simulink model "MotorControlLibNEWFixedP_FULL19b"  (R2020b)
settings: Solver=FixedStepDiscrete  StartTime=0.0  StopTime=100  FixedStep=Ts  RelTol=1e-3
values from neighbouring files (symbols this model uses):
  Ki_Iab_EMFobs = 1600.0    [MotorControl.sldd]
  Kp_Iab_EMFobs = 0.255    [MotorControl.sldd]
  p = 8/2    (= 4)    [MotorControlLibData.m]    (also in local_pmsm_torque_control_data.m = 8)
  Ts = 250.0e-06    (= 0.00025)    [MotorControlLibData.m]    (also in local_pmsm_torque_control_data.m = 5e-06)
undefined symbols (not defined in the file or in its folder): BrkPoints, CuttOffFreq_c, d_q_Voltage_Limiter_max, d_q_Voltage_Limiter_sat_neg, d_q_Voltage_Limiter_sat_pos, DiscIntNeverNeededParam, Down, dSoll, EMFobsLdGain, EMFobsRS, Ki_dAxis, Ki_qAxis, Kp_dAxis, Kp_qAxis, MaxBckEMFVol_sat_neg, MaxBckEMFVol_sat_pos, NumBits1, NumBits2, pwmTableData, qSoll, Slope1, Slope2, TqToIqConst, TsIntern, Up
libraries: simulink x13, pid_lib x6, eePwmGenerator x3, simulink_extras x2
(part 1 of 3)
settings Model: DataDictionary=MotorControl.sldd  NumberOfSteps=10  Creator=unix  LastModifiedBy=unix
settings SolverCC: AutoInsertRateTranBlk=on
settings OptimizationCC: DefaultParameterBehavior=Inlined  EnhancedBackFolding=on  PassReuseOutputArgsAs=Individual arguments  ZeroExternalMemoryAtStartup=off  ZeroInternalMemoryAtStartup=off  OptimizeBlockOrder=speed  DifferentSizesBufferReuse=on  OptimizationCustomize=off  EfficientTunableParamExpr=on
settings DebuggingCC: ArrayBoundsChecking=warning  SignalInfNanChecking=warning  SignalRangeChecking=warning  CheckMatrixSingularityMsg=warning  IntegerOverflowMsg=error  ParameterOverflowMsg=warning  ParameterUnderflowMsg=warning  ParameterPrecisionLossMsg=none  ParameterTunabilityLossMsg=error  UnderSpecifiedDataTypeMsg=warning  IntegerSaturationMsg=error
settings SFSimCC: MATLABDynamicMemAlloc=off
settings RTWCC: Description=Embedded Coder  SystemTargetFile=ert.tlc  GenCodeOnly=on  TemplateMakefile=ert_default_tmf  GenerateReport=on  IncludeHyperlinkInReport=on  LaunchReport=on  GenerateTraceInfo=on  GenerateTraceReport=on  GenerateTraceReportSl=on  GenerateTraceReportSf=on  GenerateTraceReportEml=on
settings CodeAppCC: ForceParamTrailComments=on  IgnoreCustomStorageClasses=off  OperatorAnnotations=on  SimulinkDataObjDesc=on  SFDataObjDesc=on  InsertBlockDesc=on
settings ERTTargetCC: TargetLangStandard=C99 (ISO)  GenerateSampleERTMain=on  GenerateASAP2=on  InlinedParameterPlacement=NonHierarchical  ERTCustomFileTemplate=example_file_process.tlc

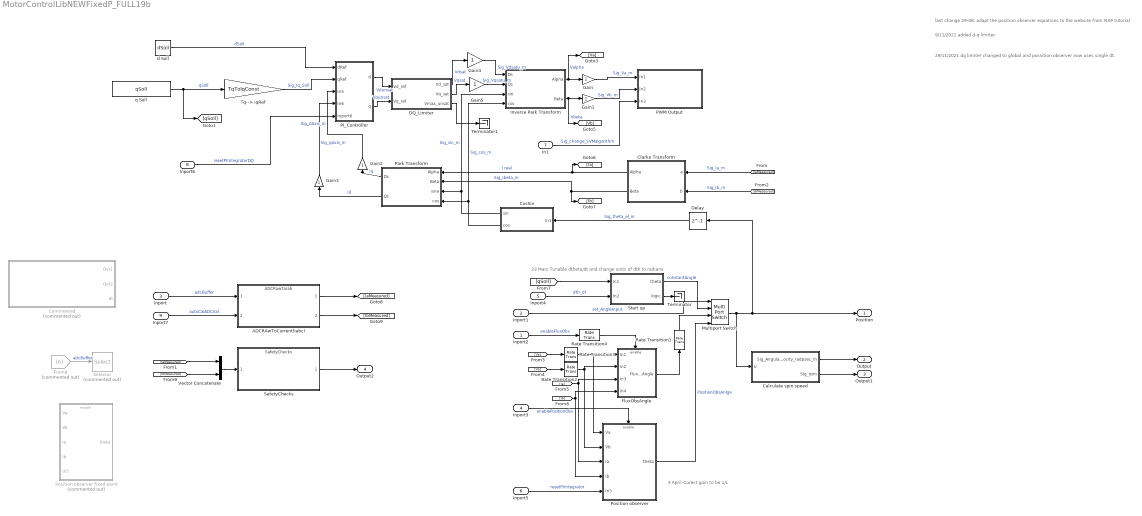
== system MotorControlLibNEWFixedP_FULL19b ==
  note: 29/11/2021 dq limiter changed to global and possition observer now uses single dt.
  note: 9/11/2021 added d-q limiter.
  note: last change 29-08: adapt the position observer equations to the website from NXP tutorial
  note: 3 April-Corect gain to be 1/L
  note: 23 Marz Tunable dtheta/dt and change units of dth to radians
  Inport2 : Inport  OutDataTypeStr=boolean  SampleTime=4*Ts
      settings: AttributesFormatString=%<SampleTime>
  Inport1 : Inport  Port=2  OutDataTypeStr=uint8  SampleTime=4*Ts
      settings: AttributesFormatString=%<SampleTime>
  Inport : Inport  Port=3
  Inport3 : Inport  Port=4  OutDataTypeStr=boolean  SampleTime=4*Ts
      settings: AttributesFormatString=%<SampleTime>
  Inport4 : Inport  Port=5
  Inport5 : Inport  Port=6  OutDataTypeStr=boolean  SampleTime=4*Ts
      settings: AttributesFormatString=%<SampleTime>
  In1 : Inport  Port=7
  Inport6 : Inport  Port=8  OutDataTypeStr=boolean
  Inport7 : Inport  Port=9
  ADCRAwToCurrent(Iabc) : ModelReference  ModelNameDialog=ADCRawToIab  ModelReferenceVersion=3.5
  Calculate spin speed : Subsystem  TreatAsAtomicUnit=on  SystemSampleTime=4*Ts
  Clarke Transform : Subsystem  VariantControl=Variant2  mask(Clarke Transform){}
      mask help:
      | <p>Compute Clarke transformation on balanced 3-phase inputs into balanced 2-phase orthogonal outputs.
      | <br>
      | <br>
      | The block accepts two signals out of three phases, and outputs corresponding &alpha;-&beta; axis components, where phase-a axis is aligned with alpha axis.</p>
      mask Help: eval('mcb.internal.helpview(''clarketransform'')')
      mask Display: mcb.internal.drawIcons('Clarke',1);
  Commented : Subsystem  Commented=on
  CosSin : Subsystem
  DQ_Limiter : Subsystem  TreatAsAtomicUnit=on  SystemSampleTime=4*Ts  mask(DQ Limiter){Vmax=d_q_Voltage_Limiter_max}
      mask prompts: Vmax "D-Q saturation limit:"
      mask help:
      | Implement saturation on reference dq voltages, with respect to phase voltage peak limit.
      |
      | The block accepts reference values of d and q axis voltages, and outputs corresponding saturated values along with unsaturated peak value to initiate field weakening control.
      |
      | Enter the phase voltage peak limit in the dialog box to initiate saturation.
      settings: RTWFcnNameOpts=Use subsystem name
      mask Help: eval('mcb.internal.helpview(''dqlimiter'')')
  Delay : Delay  DelayLength=1  SampleTime=4*Ts
      settings: AttributesFormatString=%<SampleTime>
  FluxObsAngle : Subsystem
      settings: RTWFcnNameOpts=Use subsystem name
  From8 : From  Commented=on
  Gain{,1..3} (4 alike) : Gain  OutDataTypeStr=Inherit: Same as input  ParamDataTypeStr=Inherit: Same as input
  Gain4 : Gain  OutDataTypeStr=Inherit: Inherit via back propagation
  Gain5 : Gain  OutDataTypeStr=Inherit: Inherit via back propagation
  Inverse Park Transform : Subsystem  SystemSampleTime=250*Ts  mask(Inverse Park Transform){AxisAlignment=D-axis}
      mask prompts: AxisAlignment "Alpha (phase-a) axis alignment:"
      mask help:
      | <p>Compute Inverse Park transformation on rotating reference frame inputs into stationary reference frame outputs.
      | <br><br>
      | The block accepts the following:
      | <ul>
      | <li>d-q axis components in rotating reference frame</li>
      | <li>Sine and cosine values of corresponding angle of transformation</li>
      | </ul>
      | The block outputs &alpha;-&beta; axis components in stationary reference frame.
      | <br><br>
      | D-axis alignment with alpha (phase-a) is popular in motor control theory while Q-axis alignment with alpha (phase-a) is more suitable for power conversion applications.</p>
      mask Help: eval('mcb.internal.helpview(''inverseparktransform'')')
      mask TypeOptions AxisAlignment: D-axis | Q-axis
  Multiport Switch : MultiPortSwitch  DataPortOrder=Zero-based contiguous  zeroidx=on
  PI_Controller : Subsystem  TreatAsAtomicUnit=on  SystemSampleTime=4*Ts
      settings: RTWFcnNameOpts=Use subsystem name
  PWM Output : Subsystem
  Park Transform : Subsystem  SystemSampleTime=250*Ts  mask(Park Transform){AxisAlignment=D-axis}
      mask prompts: AxisAlignment "Alpha (phase-a) axis alignment:"
      mask help:
      | <p>Compute Park transformation on stationary reference frame inputs into rotating reference frame outputs.
      | <br><br>
      | The block accepts the following:
      | <ul>
      |   <li>&alpha;-&beta; axis components in stationary reference frame</li>
      |   <li>Sine and cosine values of corresponding angle of transformation</li>
      | </ul>
      | The block outputs direct and quadrature axis components in rotating reference frame.
      | <br><br>
      | D-axis alignment with alpha (phase-a) is popular in motor control theory while Q-axis alignment with alpha (phase-a) is more suitable for power conversion applications.</p>
      mask Help: eval('mcb.internal.helpview(''parktransform'')')
      mask TypeOptions AxisAlignment: D-axis | Q-axis
      mask Display: mcb.internal.drawIcons('Park',1);
  Position observer : Subsystem
  Position observer fixed point : Subsystem  Commented=on
  Rate Transition{1..4} (4 alike) : RateTransition
  SafetyChecks : ModelReference  ModelNameDialog=SafetyChecks.slx  ModelReferenceVersion=1.11
  Selector : Selector  Commented=on  InputPortWidth=3  IndexOptions=Index vector (dialog)  Indices=[1 2]  OutputSizes=1
  Start up : Subsystem  TreatAsAtomicUnit=on  SystemSampleTime=4*Ts
  Terminator : Terminator
  Terminator1 : Terminator
  Tq--> iqRef : Gain  Gain=TqToIqConst  ParamDataTypeStr=Inherit: Inherit from 'Gain'  OutDataTypeStr=fixdt(1,16,2^-8,0)
  Vector Concatenate : Concatenate
  d Soll : Constant  Value=dSoll
  q Soll : Constant  Value=qSoll
  Position : Outport
  Output : Outport  Port=2
  Output1 : Outport  Port=3  Unit=rpm
  Output2 : Outport  Port=4
  wires:
  [IbMeasured] -> Clarke Transform/2(b)  "Sig_Ib_m"
  [IaMeasured] -> Clarke Transform/1(a)  "Sig_Ia_m"
  Clarke Transform/1(Alpha) -> [Ia], Park Transform/1(Alpha)  "I real"
  Clarke Transform/2(Beta) -> [Ib], Park Transform/2(Beta)  "Sig_Ibeta_m"
  Inverse Park Transform/1(Alpha) -> [Va], Gain/1  "Valpha"
  Gain4/1 -> Inverse Park Transform/1(Ds)  "Sig_Vdsatu_m"
  Gain5/1 -> Inverse Park Transform/2(Qs)  "Sig_Vqsatu_m"
  Inverse Park Transform/2(Beta) -> Gain1/1, [Vb]  "Vbeta"
  d Soll/1 -> PI_Controller/1(dRef)  "dSoll"
  Tq--> iqRef/1 -> PI_Controller/2(qRef)  "Sig_Iq_Soll"
  PI_Controller/1(d) -> DQ_Limiter/1(Vd_ref)  "Vdunsat"
  PI_Controller/2(q) -> DQ_Limiter/2(Vq_ref)  "Vqunsat"
  Park Transform/2(Qs) -> Gain3/1  "Id"
  Park Transform/1(Ds) -> Gain2/1  "Iq"
  q Soll/1 -> [qSoll], Tq--> iqRef/1  "qSoll"
  ADCRAwToCurrent(Iabc)/2 -> [IbMeasured]
  Inport/1 -> ADCRAwToCurrent(Iabc)/1  "adcBuffer"
  ADCRAwToCurrent(Iabc)/1 -> [IaMeasured]
  CosSin/1(sin) -> Inverse Park Transform/3(sin), Park Transform/3(sine)  "Sig_sin_m"
  CosSin/2(cos) -> Park Transform/4(cos), Inverse Park Transform/4(cos)  "Sig_cos_m"
  Delay/1 -> CosSin/1(In1)  "Sig_theta_el_m"
  Gain/1 -> PWM Output/1(In1)  "Sig_Va_m"
  Gain1/1 -> PWM Output/2(In2)  "Sig_Vb_m"
  Gain2/1 -> PI_Controller/3(In5)  "Sig_dAxis_m"
  Gain3/1 -> PI_Controller/4(In6)  "Sig_qAxis_m"
  [qSoll] -> Start up/1(In1)
  Start up/1(theta) -> Multiport Switch/2  "constantAngle"
  Start up/2(logic) -> Terminator/1
  Inport1/1 -> Multiport Switch/1  "set_AngleInput"
  FluxObsAngle/1(FluxObsAngle) -> Rate Transition1/1
  Inport2/1 -> Rate Transition4/1  "enableFluxObs"
  Inport3/1 -> Position observer/Enable  "enablePositionObs"
  Position observer/1(theta) -> Multiport Switch/4  "PositionObsAnlge"
  Rate Transition2/1 -> FluxObsAngle/2(In2), Position observer/2(Vb)
  Rate Transition3/1 -> Position observer/1(Va), FluxObsAngle/1(In1)
  [Ia] -> FluxObsAngle/3(In3), Position observer/3(Ia)
  [Ib] -> FluxObsAngle/4(In4), Position observer/4(Ib)
  From8/1 -> Selector/1  "adcBuffer"
  Inport4/1 -> Start up/2(In2)  "dth_dt"
  Inport5/1 -> Position observer/5(In5)  "resetPIIntegrator"
  DQ_Limiter/2(Vq_sat) -> Gain5/1  "Vqsat"
  DQ_Limiter/1(Vd_sat) -> Gain4/1  "Vdsat"
  DQ_Limiter/3(Vmax_unsat) -> Terminator1/1
  Rate Transition4/1 -> FluxObsAngle/Enable
  In1/1 -> PWM Output/3(In3)  "Sig_change_SVMalgorithm"
  Multiport Switch/1 -> Calculate spin speed/1(U), Delay/1, Position/1
  Inport6/1 -> PI_Controller/5(Inport6)  "resetPIIntegratorDQ"
  Rate Transition1/1 -> Multiport Switch/3
  [Vb] -> Rate Transition2/1
  [Va] -> Rate Transition3/1
  Calculate spin speed/1(Sig_Angular_Velocity_radpsec_m) -> Output/1
  Calculate spin speed/2(Sig_rpm) -> Output1/1
  Vector Concatenate/1 -> SafetyChecks/1
  [IaMeasured] -> Vector Concatenate/1
  [IbMeasured] -> Vector Concatenate/2
  SafetyChecks/1 -> Output2/1
  Inport7/1 -> ADCRAwToCurrent(Iabc)/2  "autoCalADCVal"

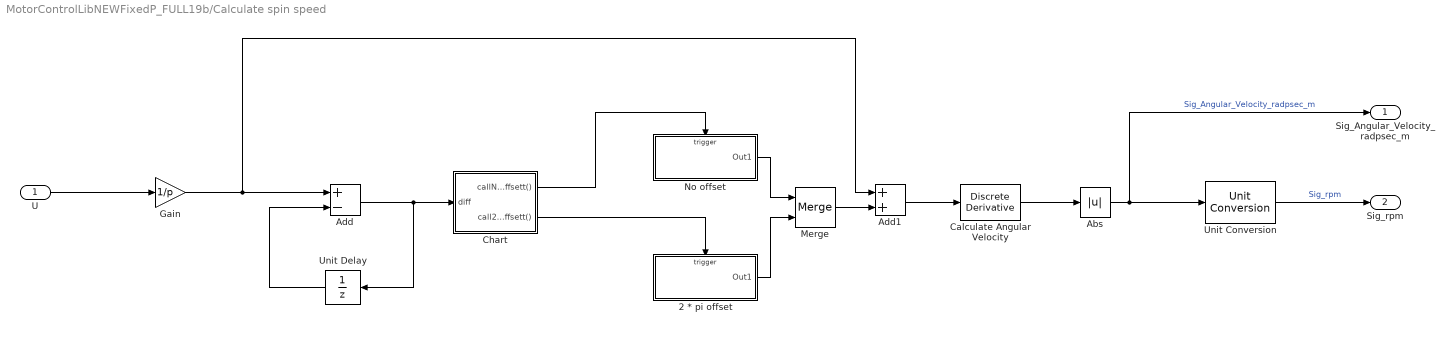
== system MotorControlLibNEWFixedP_FULL19b/Calculate spin speed ==
  U : Inport
  2 * pi offset : Subsystem  TreatAsAtomicUnit=on
  Abs : Abs
  Add : Sum  Inputs=+-
  Add1 : Sum
  Calculate Angular Velocity : simulink/Discrete/Discrete Derivative  gainval=1.0  ICPrevScaledInput=0.0  OutMin=[]  OutMax=[]  OutDataTypeStr=single  OutputDataTypeScalingMode=single  OutDataType=fixdt(1, 16)  OutScaling=2^-10  DoSatur=off
  Chart : Stateflow chart  TreatAsAtomicUnit=on
  Gain : Gain  Gain=1/p  OutDataTypeStr=single
  Merge : Merge
  No offset : Subsystem  TreatAsAtomicUnit=on
  Unit Conversion : UnitConversion
  Unit Delay : UnitDelay  SampleTime=-1  HasFrameUpgradeWarning=on
  Sig_Angular_Velocity_radpsec_m : Outport
  Sig_rpm : Outport  Port=2
  wires:
  U/1 -> Gain/1
  Unit Conversion/1 -> Sig_rpm/1  "Sig_rpm"
  Abs/1 -> Unit Conversion/1, Sig_Angular_Velocity_radpsec_m/1  "Sig_Angular_Velocity_radpsec_m"
  Calculate Angular Velocity/1 -> Abs/1
  Unit Delay/1 -> Add/2
  Add/1 -> Unit Delay/1, Chart/1(diff)
  Chart/2(call2PiOffsett()) -> 2 * pi offset/Trigger
  Chart/1(callNoOffsett()) -> No offset/Trigger
  2 * pi offset/1(Out1) -> Merge/2
  No offset/1(Out1) -> Merge/1
  Merge/1 -> Add1/2
  Add1/1 -> Calculate Angular Velocity/1
  Gain/1 -> Add1/1, Add/1

== system MotorControlLibNEWFixedP_FULL19b/Clarke Transform ==
  a : Inport
  b : Inport  Port=2
  Data Type Duplicate : DataTypeDuplicate
  a_plus_2b : Sum  Inputs=+++  RndMeth=Simplest  OutDataTypeStr=Inherit: Same as first input
  one_by_sqrt3 : Gain  Gain=1/sqrt(3)  RndMeth=Simplest  OutDataTypeStr=Inherit: Same as input
  Alpha : Outport  VectorParamsAs1DForOutWhenUnconnected=off
  Beta : Outport  Port=2  VectorParamsAs1DForOutWhenUnconnected=off
  wires:
  a/1 -> a_plus_2b/1, Alpha/1, Data Type Duplicate/1
  one_by_sqrt3/1 -> Beta/1
  a_plus_2b/1 -> one_by_sqrt3/1
  b/1 -> a_plus_2b/2, a_plus_2b/3, Data Type Duplicate/2

== system MotorControlLibNEWFixedP_FULL19b/Commented ==
  Digital Clock : DigitalClock  Commented=on  SampleTime=Ts
  Function-Call Clock_50us : simulink/Ports & Subsystems/Function-Call Generator  Commented=on  sample_time=5e-5  numberOfIterations=1  DisallowWideOutput=off
  Function-Call Clock_50us1 : simulink/Ports & Subsystems/Function-Call Generator  Commented=on  sample_time=Ts  numberOfIterations=1  DisallowWideOutput=off
  Function-Call Split : FunctionCallSplit  Commented=on  IconShape=distinctive  NumOutputPorts=3  OutputPortLayout=default
  Goto1 : Goto  Commented=on  GotoTag=Task100us_2
  Goto2 : Goto  Commented=on  GotoTag=Task100us_1
  Goto4 : Goto  Commented=on  GotoTag=Task1ms_1
  Rate Transition8 : RateTransition  Commented=on
  Subsystem : Subsystem  Commented=on
  Task Scheduler : Stateflow chart  Commented=on  TreatAsAtomicUnit=on
  Out1 : Outport
  Out2 : Outport  Port=2
  dt : Outport  Port=3
  wires:
  Task Scheduler/2(Task_100us_2()) -> Goto1/1
  Function-Call Clock_50us/1 -> Task Scheduler/Trigger
  Digital Clock/1 -> Rate Transition8/1
  Rate Transition8/1 -> Subsystem/1(Clock)
  Function-Call Clock_50us1/1 -> Function-Call Split/1
  Function-Call Split/3 -> Subsystem/Trigger
  Subsystem/1(dt) -> dt/1
  Function-Call Split/2 -> Out2/1
  Function-Call Split/1 -> Out1/1
  Task Scheduler/1(Task_100us_1()) -> Goto2/1
  Task Scheduler/3(Task_1ms_1()) -> Goto4/1

== system MotorControlLibNEWFixedP_FULL19b/CosSin ==
  In1 : Inport
  Data Type Conversion1 : DataTypeConversion
  Sine-Cosine Lookup : Subsystem  mask(Sine-Cosine Lookup){AngleInput=Radians, N_points=512}
      mask prompts: AngleInput "Theta units:"; N_points "Number of data points for lookup table:"
      mask help:
      | Implement sine and cosine functions using a lookup table approach for optimized performance on target hardware.
      |
      | The block accepts input angle in different units and outputs corresponding sine and cosine values.
      mask init:
      | % dlgSett = mct.internal.SinCosCb(gcbh);
      | this = get_param(gcbh,'Object');
      | 
      | points = eval(this.N_points);
      | 
      | dlgSett.points = 125*floor(points/125);
      | 
      | dlgSett.Offset = uint16(dlgSett.points/5);
      | 
      | dlgSett.N_points = 4*dlgSett.Offset;
      | N_points = dlgSett.N_points;
      | 
      | theta = linspace(0,2*pi,N_points+1);
      | dlgSett.size = 5*dlgSett.Offset+2;
      | dlgSett.sin_table = zeros(1,dlgSett.size);
      | dlgSett.sin_table(1:N_points+1) = sin(theta);
      | dlgSett.sin_table(N_points+2:dlgSett.size) = dlgSett.sin_table(2:0.25*N_points+2);
      | 
      | dlgSett.N_points = double(dlgSett.N_points);
      | dlgSett.index_gain = dlgSett.N_points;
      | dlgSett.UpperSatLimit = 1;
      | 
      | switch AngleInput
      |     case 1
      |         dlgSett.UpperSatLimit = 1;
      |     case 2
      |         dlgSett.UpperSatLimit = 2*pi;
      |     case 3
      |         dlgSett.UpperSatLimit = 360;
      |     otherwise
      | end
      mask Help: eval('mcb.internal.helpview(''sinecosinelookup'')')
      mask TypeOptions AngleInput: Per-unit | Radians | Degrees
      mask Display: mcb.internal.drawIcons('Sin-Cos',1);
  sin : Outport
  cos : Outport  Port=2
  wires:
  Sine-Cosine Lookup/2(cos) -> cos/1
  In1/1 -> Data Type Conversion1/1
  Sine-Cosine Lookup/1(sin) -> sin/1
  Data Type Conversion1/1 -> Sine-Cosine Lookup/1(Theta)

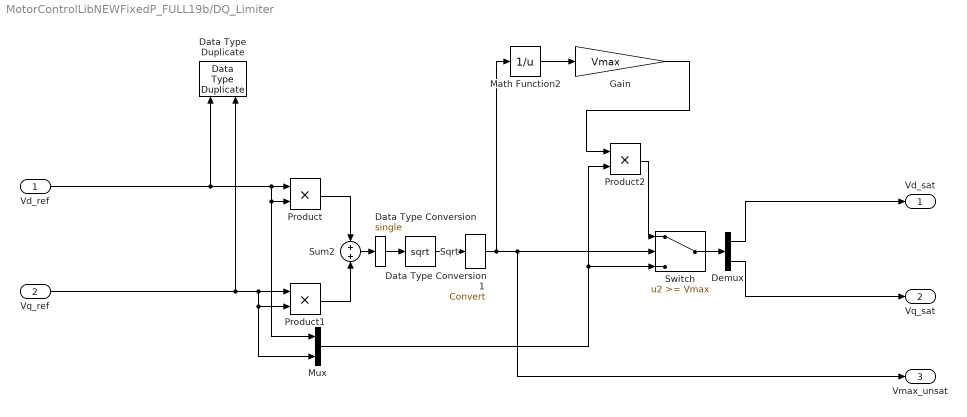
== system MotorControlLibNEWFixedP_FULL19b/DQ_Limiter ==
  Vd_ref : Inport
  Vq_ref : Inport  Port=2
  Data Type Duplicate : DataTypeDuplicate
  Data Type Conversion : DataTypeConversion  OutDataTypeStr=single
  Data Type Conversion1 : DataTypeConversion
  Demux : Demux  Outputs=2
  Gain : Gain  Gain=Vmax  OutDataTypeStr=Inherit: Same as input
  Math Function2 : Math  Operator=reciprocal  SignedPower=on  RndMeth=Simplest
  Mux : Mux  Inputs=2
  Product : Product  RndMeth=Simplest  OutDataTypeStr=Inherit: Same as first input
  Product1 : Product  RndMeth=Simplest  OutDataTypeStr=Inherit: Same as first input
  Product2 : Product  OutDataTypeStr=Inherit: Same as first input
  Sqrt : Sqrt  IntermediateResultsDataTypeStr=Inherit: Inherit from input  SaturateOnIntegerOverflow=on
  Sum2 : Sum  OutDataTypeStr=Inherit: Same as first input
  Switch : Switch  Threshold=Vmax  ZeroCross=off
  Vd_sat : Outport  VectorParamsAs1DForOutWhenUnconnected=off
  Vq_sat : Outport  Port=2  VectorParamsAs1DForOutWhenUnconnected=off
  Vmax_unsat : Outport  Port=3  VectorParamsAs1DForOutWhenUnconnected=off
  wires:
  Vd_ref/1 -> Data Type Duplicate/1, Product/1, Product/2, Mux/1
  Demux/1 -> Vd_sat/1
  Product1/1 -> Sum2/2
  Product/1 -> Sum2/1
  Sum2/1 -> Data Type Conversion/1
  Math Function2/1 -> Gain/1
  Mux/1 -> Product2/2, Switch/3
  Product2/1 -> Switch/1
  Switch/1 -> Demux/1
  Demux/2 -> Vq_sat/1
  Sqrt/1 -> Data Type Conversion1/1
  Gain/1 -> Product2/1
  Vq_ref/1 -> Data Type Duplicate/2, Product1/1, Product1/2, Mux/2
  Data Type Conversion1/1 -> Vmax_unsat/1, Switch/2, Math Function2/1
  Data Type Conversion/1 -> Sqrt/1

== system MotorControlLibNEWFixedP_FULL19b/FluxObsAngle ==
  In1 : Inport
  In2 : Inport  Port=2
  In3 : Inport  Port=3
  In4 : Inport  Port=4
  Enable : EnablePort
  Flux Observer : Subsystem  TreatAsAtomicUnit=on  SystemSampleTime=2*Ts  mask(Flux Observer){BlockInputUnit=SI unit, PerUnitVoltage=13.86, PerUnitCurrent=19.3, PositionSelect=on, FluxSelect=off, TorqueSelect=off, PolePairs=4, StatorResistance=EMFobsRS, StatorDAxisInductance=EMFobsLdGain, BlockSampleTime=2*Ts, PositionUnit=Radians, PositionDatatype=fixdt(1,16,2^-8,0), FluxUnit=Weber, PerUnitFlux=0.1, FluxDatatype=single, TorqueUnit=Nm, PerUnitTorque=100, TorqueDatatype=single}
      mask prompts: BlockInputUnit "Input units:"; PerUnitVoltage "Per unit reference voltage (V):"; PerUnitCurrent "Per unit reference current (A):"; PositionSelect "Position"; FluxSelect "Flux"; TorqueSelect "Torque"; PolePairs "Pole pairs:"; StatorResistance "Stator resistance (ohm):"; StatorDAxisInductance "Stator d-axis inductance (H):"; BlockSampleTime "Block sample time (S):"; PositionUnit "Position unit:"; PositionDatatype "Position datatype:"; FluxUnit "Flux unit:"; PerUnitFlux "Per unit flux (Wb):"; FluxDatatype "Flux datatype:"; TorqueUnit "Torque unit:"; PerUnitTorque "Per unit torque (Nm):"; TorqueDatatype "Torque datatype:"
      mask help:
      | <p>Compute &#952;<sub>e</sub> (electrical position), &#936; (magnetic flux), and T<sub>e</sub> (electrical torque) of a PMSM from the measured voltage and current in the stationary reference frame.
      | <br><br>
      | Use the Input units parameter to select the input unit of the block.
      | <br><br>
      | Use the Per unit reference voltage parameter to enter the amplitude of line-to-neutral voltage used as a reference. Use the Per unit reference current parameter to enter the amplitude of line current used as a reference.</P>
      mask init:
      | %mcb.internal.FOCb('MaskInitFcn', gcbh);
      mask Help: eval('mcb.internal.helpview(''fluxobserver'')')
      mask TypeOptions BlockInputUnit: SI unit | Per-unit
      mask Callback BlockInputUnit: mcb.internal.FOCb('MaskDisplay', gcbh);
      mask Callback PositionSelect: mcb.internal.FOCb('MaskDisplay', gcbh);
      mask Callback FluxSelect: mcb.internal.FOCb('MaskDisplay', gcbh);
      mask Callback TorqueSelect: mcb.internal.FOCb('MaskDisplay', gcbh);
      mask TypeOptions PositionUnit: Radians | Degrees | Per-unit
      mask TypeOptions FluxUnit: Weber | Per-unit
      mask Callback FluxUnit: mcb.internal.FOCb('MaskDisplay', gcbh);
      mask TypeOptions TorqueUnit: Nm | Per-unit
      mask Callback TorqueUnit: mcb.internal.FOCb('MaskDisplay', gcbh);
      mask DialogControl Container4 Prompt: Motor Parameters
      mask DialogControl Container7 Prompt: Block Output
      mask DialogControl Container8 Prompt: Datatypes
      mask Display:
      | color('black');
      | port_label('input',1, 'V_{\alpha}', 'interpreter', 'tex');
      | port_label('input',2, 'V_{\beta}', 'interpreter', 'tex');
      | port_label('input',3, 'I_{\alpha}', 'interpreter', 'tex');
      | port_label('input',4, 'I_{\beta}', 'interpreter', 'tex');
      | port_label('input',5, 'Rst', 'interpreter', 'tex');
      | port_label('output',1, '\theta_{e}', 'interpreter', 'tex');
      | %No Flux;
      | %No Torque;
      | fprintf('Flux\nObserver');
  Ground : Ground
  FluxObsAngle : Outport
  wires:
  In1/1 -> Flux Observer/1(Valpha)
  Ground/1 -> Flux Observer/5(Reset)
  In4/1 -> Flux Observer/4(Ibeta)
  In2/1 -> Flux Observer/2(Vbeta)
  In3/1 -> Flux Observer/3(Ialpha)
  Flux Observer/1(Position) -> FluxObsAngle/1  "FluxObsAngle"

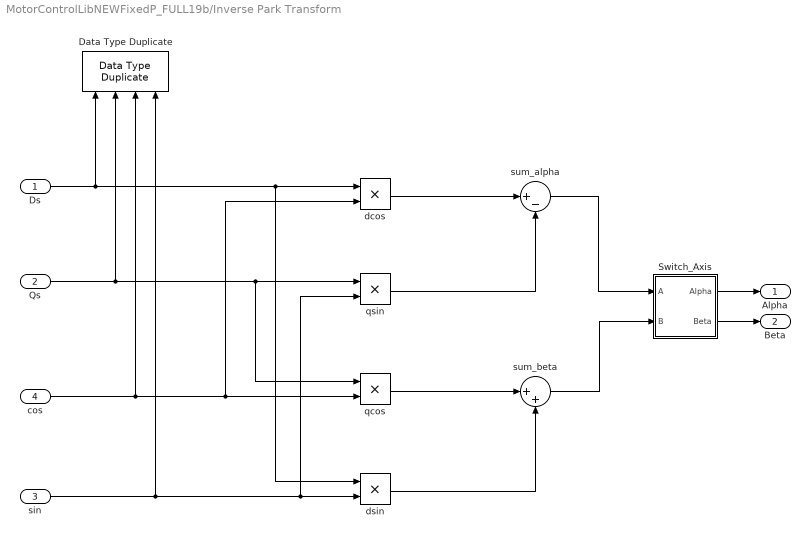
== system MotorControlLibNEWFixedP_FULL19b/Inverse Park Transform ==
  Ds : Inport
  Qs : Inport  Port=2
  sin : Inport  Port=3
  cos : Inport  Port=4
  Data Type Duplicate : DataTypeDuplicate  NumInputPorts=4
  Switch_Axis : Subsystem
  dcos : Product  RndMeth=Simplest  OutDataTypeStr=Inherit: Same as first input
  dsin : Product  RndMeth=Simplest  OutDataTypeStr=Inherit: Same as first input
  qcos : Product  RndMeth=Simplest  OutDataTypeStr=Inherit: Same as first input
  qsin : Product  RndMeth=Simplest  OutDataTypeStr=Inherit: Same as first input
  sum_alpha : Sum  Inputs=|+-  RndMeth=Simplest  OutDataTypeStr=Inherit: Same as first input
  sum_beta : Sum  Inputs=|++  RndMeth=Simplest  OutDataTypeStr=Inherit: Same as first input
  Alpha : Outport  VectorParamsAs1DForOutWhenUnconnected=off
  Beta : Outport  Port=2  VectorParamsAs1DForOutWhenUnconnected=off
  wires:
  Switch_Axis/2(Beta) -> Beta/1
  Switch_Axis/1(Alpha) -> Alpha/1
  sum_beta/1 -> Switch_Axis/2(B)
  sum_alpha/1 -> Switch_Axis/1(A)
  sin/1 -> dsin/2, qsin/2, Data Type Duplicate/4
  cos/1 -> qcos/2, dcos/2, Data Type Duplicate/3
  dsin/1 -> sum_beta/2
  Qs/1 -> qsin/1, qcos/1, Data Type Duplicate/2
  dcos/1 -> sum_alpha/1
  qcos/1 -> sum_beta/1
  qsin/1 -> sum_alpha/2
  Ds/1 -> dcos/1, dsin/1, Data Type Duplicate/1

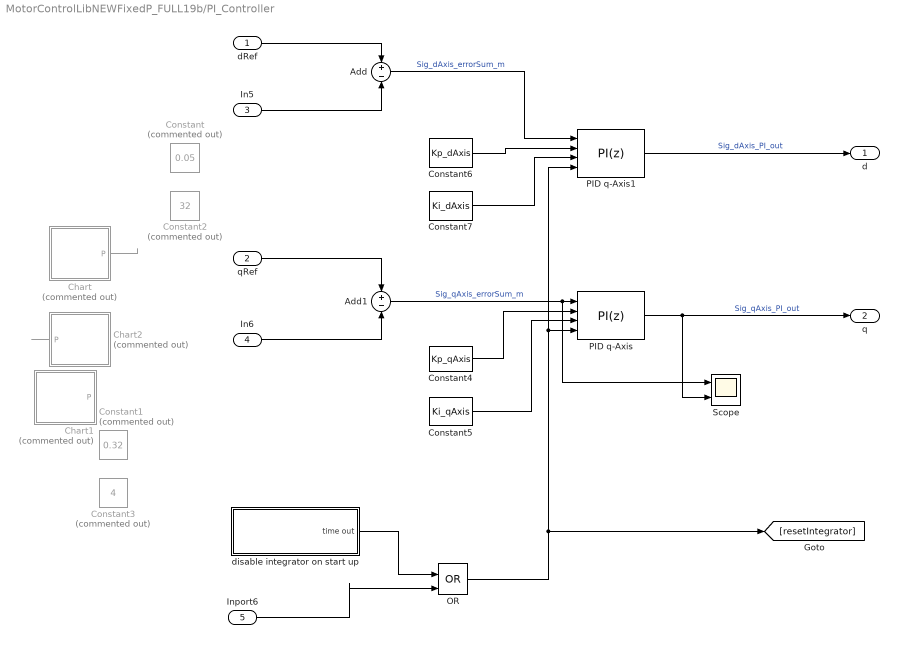
== system MotorControlLibNEWFixedP_FULL19b/PI_Controller ==
  dRef : Inport
  qRef : Inport  Port=2
  In5 : Inport  Port=3
  In6 : Inport  Port=4
  Inport6 : Inport  Port=5
  Add : Sum  Inputs=+|-
  Add1 : Sum  Inputs=+|-
  Chart : Stateflow chart  Commented=on  TreatAsAtomicUnit=on  SystemSampleTime=1000*Ts
  Chart1 : Stateflow chart  Commented=on  TreatAsAtomicUnit=on  SystemSampleTime=2000*Ts
  Chart2 : Stateflow chart  Commented=on  TreatAsAtomicUnit=on  SystemSampleTime=100000*Ts
  Constant : Constant  Commented=on  Value=0.05  OutDataTypeStr=fixdt(1,16,2^-7,0)
  Constant1 : Constant  Commented=on  Value=0.32  OutDataTypeStr=fixdt(1,8,2^-7,0)
  Constant2 : Constant  Commented=on  Value=32  OutDataTypeStr=fixdt(1,8,2^-1,0)
  Constant3 : Constant  Commented=on  Value=4  OutDataTypeStr=fixdt(1,8,2^-1,0)
  Constant4 : Constant  Value=Kp_qAxis
  Constant5 : Constant  Value=Ki_qAxis
  Constant6 : Constant  Value=Kp_dAxis
  Constant7 : Constant  Value=Ki_dAxis
  OR : Logic  Operator=OR  IconShape=distinctive  AllPortsSameDT=off  OutDataTypeStr=boolean
  PID q-Axis : pid_lib/PID Controller  Controller=PI  Form=Parallel  TimeDomain=Discrete-time  UseExternalTs=off  SampleTime=-1  IntegratorMethod=Forward Euler  FilterMethod=Forward Euler  ControllerParametersSource=external  P=0  I=0  D=0  UseFilter=on  N=100  TunerSelectOption=Transfer Function Based (PID Tuner App)  InitialConditionSource=internal  InitialConditionForIntegrator=0  InitialConditionForFilter=0  DifferentiatorICPrevScaledInput=0  ExternalReset=level  TrackingMode=off  Kt=1  LimitOutput=on  SatLimitsSource=internal  UpperSaturationLimit=d_q_Voltage_Limiter_sat_pos  LowerSaturationLimit=d_q_Voltage_Limiter_sat_neg  LinearizeAsGain=off  AntiWindupMode=clamping  Kb=10  PGainOutDataTypeStr=fixdt(1,16,2^-8,0)  PProdOutDataTypeStr=fixdt(1,16,2^-8,0)  POutMin=[]  POutMax=[]  IGainOutDataTypeStr=fixdt(1,16,2^-8,0)  IProdOutDataTypeStr=fixdt(1,16,2^-8,0)  IOutMin=[]  IOutMax=[]  DOutMin=[]  DOutMax=[]  NOutMin=[]  NOutMax=[]  SumOutDataTypeStr=fixdt(1,16,2^-8,0)  SumOutMin=[]  SumOutMax=[]  SaturationOutMin=[]  SaturationOutMax=[]  PParamMin=[]  PParamMax=[]  IParamMin=[]  IParamMax=[]  DParamMin=[]  DParamMax=[]  NParamMin=[]  NParamMax=[]  KbParamMin=[]  KbParamMax=[]  KtParamMin=[]  KtParamMax=[]  KbOutMin=[]  KbOutMax=[]  KtOutMin=[]  KtOutMax=[]  IntegratorOutDataTypeStr=fixdt(1,16,2^-8,0)  IntegratorOutMin=[]  IntegratorOutMax=[]  FilterOutMin=[]  FilterOutMax=[]  SumI1OutMin=[]  SumI1OutMax=[]  SumI2OutMin=[]  SumI2OutMax=[]  SumI3OutMin=[]  SumI3OutMax=[]  SumI4OutMin=[]  SumI4OutMax=[]  SumDOutMin=[]  SumDOutMax=[]  SumAccumDataTypeStr=fixdt(1,16,2^-8,0)  DifferentiatorOutMin=[]  DifferentiatorOutMax=[]  FilterDiffOutCoefMin=[]  FilterDiffOutCoefMax=[]  ReciprocalOutMin=[]  ReciprocalOutMax=[]  SumDenOutMin=[]  SumDenOutMax=[]  SumNumOutMin=[]  SumNumOutMax=[]  DivideOutMin=[]  DivideOutMax=[]  UdiffTsProdOutMin=[]  UdiffTsProdOutMax=[]  NTsProdOutMin=[]  NTsProdOutMax=[]  UintegralTsProdOutMin=[]  UintegralTsProdOutMax=[]  UngainTsProdOutMin=[]  UngainTsProdOutMax=[]  IntegratorContinuousStateAttributes=''  IntegratorStateMustResolveToSignalObject=off  IntegratorRTWStateStorageClass=Auto  FilterContinuousStateAttributes=''  FilterStateMustResolveToSignalObject=off  FilterRTWStateStorageClass=Auto  ParallelPVariant=ExternalParameters  IdealPVariant=Disabled  IVariant=ExternalParameters  DVariant=Disabled  IntegratorVariant=Discrete  SatVariant=Enabled  AWVariant=DiscClampingParallel  PCopyVariant=Disabled  TRVariant=Disabled  FdbkBlocksVariant=Forward  IdealPFdbkVariant=Disabled  SatFdbkVariant=Disabled  DerivativeFilterVariant=Disabled  NVariant=Disabled  NCopyVariant=Disabled_SignalSpec  FilterICVariant=Disabled  IntegratorICVariant=InternalICs  ExternalResetVariant=ExternalReset  TRSumVariant=Passthrough  SumFdbkVariant=Disabled  SumVariant=Sum_PI  TsampFilterVariant=InternalTs  TsampNgainVariant=Passthrough  TsampIntegralVariant=Passthrough  ExternalSaturationOutDataTypeStr=Inherit: Same as second input
  PID q-Axis1 : pid_lib/PID Controller  Controller=PI  Form=Parallel  TimeDomain=Discrete-time  UseExternalTs=off  SampleTime=-1  IntegratorMethod=Forward Euler  FilterMethod=Forward Euler  ControllerParametersSource=external  P=0  I=0  D=0  UseFilter=on  N=100  TunerSelectOption=Transfer Function Based (PID Tuner App)  ZeroCross=off  InitialConditionSource=internal  InitialConditionForIntegrator=0  InitialConditionForFilter=0  DifferentiatorICPrevScaledInput=0  ExternalReset=level  TrackingMode=off  Kt=1  LimitOutput=on  SatLimitsSource=internal  UpperSaturationLimit=d_q_Voltage_Limiter_sat_pos  LowerSaturationLimit=d_q_Voltage_Limiter_sat_neg  LinearizeAsGain=off  AntiWindupMode=clamping  Kb=10  PGainOutDataTypeStr=fixdt(1,16,2^-8,0)  PProdOutDataTypeStr=fixdt(1,16,2^-8,0)  POutMin=[]  POutMax=[]  IGainOutDataTypeStr=fixdt(1,16,2^-8,0)  IProdOutDataTypeStr=fixdt(1,16,2^-8,0)  IOutMin=[]  IOutMax=[]  DOutMin=[]  DOutMax=[]  NOutMin=[]  NOutMax=[]  SumOutDataTypeStr=fixdt(1,16,2^-8,0)  SumOutMin=[]  SumOutMax=[]  SaturationOutMin=[]  SaturationOutMax=[]  PParamMin=[]  PParamMax=[]  IParamMin=[]  IParamMax=[]  DParamMin=[]  DParamMax=[]  NParamMin=[]  NParamMax=[]  KbParamMin=[]  KbParamMax=[]  KtParamMin=[]  KtParamMax=[]  KbOutMin=[]  KbOutMax=[]  KtOutMin=[]  KtOutMax=[]  IntegratorOutDataTypeStr=fixdt(1,16,2^-8,0)  IntegratorOutMin=[]  IntegratorOutMax=[]  FilterOutMin=[]  FilterOutMax=[]  SumI1OutMin=[]  SumI1OutMax=[]  SumI2OutMin=[]  SumI2OutMax=[]  SumI3OutMin=[]  SumI3OutMax=[]  SumI4OutMin=[]  SumI4OutMax=[]  SumDOutMin=[]  SumDOutMax=[]  SumAccumDataTypeStr=fixdt(1,16,2^-8,0)  DifferentiatorOutMin=[]  DifferentiatorOutMax=[]  FilterDiffOutCoefMin=[]  FilterDiffOutCoefMax=[]  ReciprocalOutMin=[]  ReciprocalOutMax=[]  SumDenOutMin=[]  SumDenOutMax=[]  SumNumOutMin=[]  SumNumOutMax=[]  DivideOutMin=[]  DivideOutMax=[]  UdiffTsProdOutMin=[]  UdiffTsProdOutMax=[]  NTsProdOutMin=[]  NTsProdOutMax=[]  UintegralTsProdOutMin=[]  UintegralTsProdOutMax=[]  UngainTsProdOutMin=[]  UngainTsProdOutMax=[]  IntegratorContinuousStateAttributes=''  IntegratorStateMustResolveToSignalObject=off  IntegratorRTWStateStorageClass=Auto  FilterContinuousStateAttributes=''  FilterStateMustResolveToSignalObject=off  FilterRTWStateStorageClass=Auto  ParallelPVariant=ExternalParameters  IdealPVariant=Disabled  IVariant=ExternalParameters  DVariant=Disabled  IntegratorVariant=Discrete  SatVariant=Enabled  AWVariant=DiscClampingParallel  PCopyVariant=Disabled  TRVariant=Disabled  FdbkBlocksVariant=Forward  IdealPFdbkVariant=Disabled  SatFdbkVariant=Disabled  DerivativeFilterVariant=Disabled  NVariant=Disabled  NCopyVariant=Disabled_SignalSpec  FilterICVariant=Disabled  IntegratorICVariant=InternalICs  ExternalResetVariant=ExternalReset  TRSumVariant=Passthrough  SumFdbkVariant=Disabled  SumVariant=Sum_PI  TsampFilterVariant=InternalTs  TsampNgainVariant=Passthrough  TsampIntegralVariant=Passthrough  ExternalSaturationOutDataTypeStr=Inherit: Same as second input
  Scope : Scope  NumInputPorts=2
  disable integrator on start up : Subsystem
  d : Outport
  q : Outport  Port=2
  wires:
  dRef/1 -> Add/1
  qRef/1 -> Add1/1
  In6/1 -> Add1/2
  PID q-Axis/1 -> Scope/2, q/1  "Sig_qAxis_PI_out"
  PID q-Axis1/1 -> d/1  "Sig_dAxis_PI_out"
  In5/1 -> Add/2
  Add1/1 -> Scope/1, PID q-Axis/1  "Sig_qAxis_errorSum_m"
  Chart/1(P) -> ?
  Chart2/1(P) -> ?
  Constant5/1 -> PID q-Axis/3
  Constant4/1 -> PID q-Axis/2
  Add/1 -> PID q-Axis1/1  "Sig_dAxis_errorSum_m"
  Constant6/1 -> PID q-Axis1/2
  Constant7/1 -> PID q-Axis1/3
  OR/1 -> [resetIntegrator], PID q-Axis1/4, PID q-Axis/4
  disable integrator on start up/1(time out) -> OR/1
  Inport6/1 -> OR/2

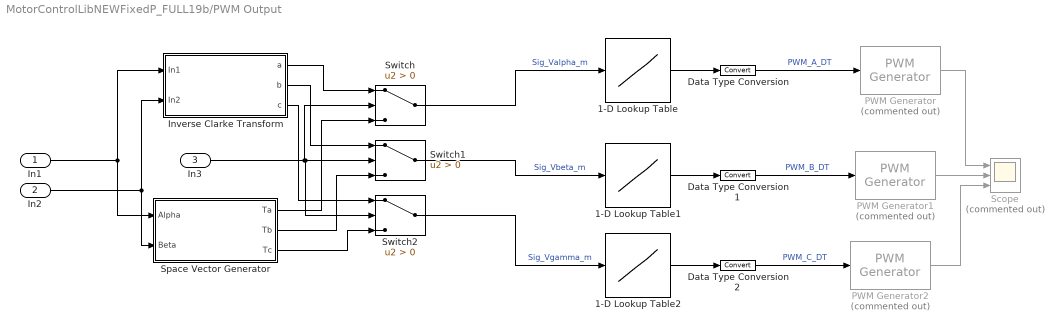
== system MotorControlLibNEWFixedP_FULL19b/PWM Output ==
  In1 : Inport
  In2 : Inport  Port=2
  In3 : Inport  Port=3
  1-D Lookup Table : Lookup_n-D  NumberOfTableDimensions=1  BreakpointsForDimension1=BrkPoints  Table=pwmTableData  ExtrapMethod=Clip  InternalRulePriority=Speed  OutDataTypeStr=uint16  RndMeth=Simplest  SaturateOnIntegerOverflow=on  InputSameDT=on
  1-D Lookup Table1 : Lookup_n-D  NumberOfTableDimensions=1  BreakpointsForDimension1=BrkPoints  Table=pwmTableData  ExtrapMethod=Clip  InternalRulePriority=Speed  OutDataTypeStr=uint16  RndMeth=Simplest  SaturateOnIntegerOverflow=on  InputSameDT=on
  1-D Lookup Table2 : Lookup_n-D  NumberOfTableDimensions=1  BreakpointsForDimension1=BrkPoints  Table=pwmTableData  ExtrapMethod=Clip  InternalRulePriority=Speed  OutDataTypeStr=uint16  RndMeth=Simplest  SaturateOnIntegerOverflow=on  InputSameDT=on
  Data Type Conversion : DataTypeConversion
  Data Type Conversion1 : DataTypeConversion
  Data Type Conversion2 : DataTypeConversion
  Inverse Clarke Transform : Subsystem  TreatAsAtomicUnit=on  mask(Inverse Clarke Transform){}
      mask help:
      | <p>Compute Inverse Clarke transformation on balanced 2-phase orthogonal inputs into balanced 3-phase outputs.
      | <br><br>
      | The block accepts &alpha;-&beta; axis components and outputs corresponding 3-phase outputs, where phase-a axis is aligned with &alpha;-axis.</p>
      mask Help: eval('mcb.internal.helpview(''inverseclarketransform'')')
      mask Display: mcb.internal.drawIcons('invClarke',1);
  PWM Generator : eePwmGenerator/PWM Generator  Commented=on  CarrCount=Up-Down  Tper=10*Ts  Ts=Ts
  PWM Generator1 : eePwmGenerator/PWM Generator  Commented=on  CarrCount=Up-Down  Tper=10*Ts  Ts=Ts
  PWM Generator2 : eePwmGenerator/PWM Generator  Commented=on  CarrCount=Up-Down  Tper=10*Ts  Ts=Ts
  Scope : Scope  Commented=on  NumInputPorts=3
  Space Vector Generator : Subsystem  TreatAsAtomicUnit=on  mask(Space Vector Generator){}
      mask help:
      | <p>Generate space vector modulation signals from stator reference voltages described by  &alpha;-&beta; components.
      | <br><br>
      | The block accepts V<sub>&alpha;</sub> and V<sub>&beta;</sub> voltages and outputs corresponding space vector modulation voltages.</p>
      mask Help: eval('mcb.internal.helpview(''spacevectorgenerator'')')
      mask Display: mcb.internal.drawIcons('SVPWM',1);
  Switch : Switch  Criteria=u2 > Threshold
  Switch1 : Switch  Criteria=u2 > Threshold
  Switch2 : Switch  Criteria=u2 > Threshold
  wires:
  In2/1 -> Space Vector Generator/2(Beta), Inverse Clarke Transform/2(In2)
  In1/1 -> Space Vector Generator/1(Alpha), Inverse Clarke Transform/1(In1)
  Switch/1 -> 1-D Lookup Table/1  "Sig_Valpha_m"
  1-D Lookup Table/1 -> Data Type Conversion/1
  Switch1/1 -> 1-D Lookup Table1/1  "Sig_Vbeta_m"
  Switch2/1 -> 1-D Lookup Table2/1  "Sig_Vgamma_m"
  PWM Generator/1 -> Scope/1
  1-D Lookup Table2/1 -> Data Type Conversion2/1
  1-D Lookup Table1/1 -> Data Type Conversion1/1
  PWM Generator1/1 -> Scope/2
  PWM Generator2/1 -> Scope/3
  Data Type Conversion/1 -> PWM Generator/1  "PWM_A_DT"
  Data Type Conversion1/1 -> PWM Generator1/1  "PWM_B_DT"
  Data Type Conversion2/1 -> PWM Generator2/1  "PWM_C_DT"
  Space Vector Generator/1(Ta) -> Switch/3
  Space Vector Generator/2(Tb) -> Switch1/3
  Space Vector Generator/3(Tc) -> Switch2/3
  Inverse Clarke Transform/1(a) -> Switch/1
  Inverse Clarke Transform/2(b) -> Switch1/1
  Inverse Clarke Transform/3(c) -> Switch2/1
  In3/1 -> Switch2/2, Switch1/2, Switch/2

== system MotorControlLibNEWFixedP_FULL19b/Park Transform ==
  Alpha : Inport
  Beta : Inport  Port=2
  sine : Inport  Port=3
  cos : Inport  Port=4
  Data Type Duplicate : DataTypeDuplicate  NumInputPorts=4
  Switch_Axis : Subsystem
  acos : Product  RndMeth=Simplest  OutDataTypeStr=Inherit: Same as first input
  asin : Product  RndMeth=Simplest  OutDataTypeStr=Inherit: Same as first input
  bcos : Product  OutDataTypeStr=Inherit: Inherit via back propagation  RndMeth=Simplest
  bsin : Product  OutDataTypeStr=Inherit: Inherit via back propagation  RndMeth=Simplest
  sum_Ds : Sum  Inputs=|++  RndMeth=Simplest  OutDataTypeStr=Inherit: Same as first input
  sum_Qs : Sum  Inputs=|+-  RndMeth=Simplest  OutDataTypeStr=Inherit: Same as first input
  Ds : Outport  VectorParamsAs1DForOutWhenUnconnected=off
  Qs : Outport  Port=2  VectorParamsAs1DForOutWhenUnconnected=off
  wires:
  Beta/1 -> Data Type Duplicate/2, bcos/1, bsin/1
  Switch_Axis/1(d_axis) -> Ds/1
  Switch_Axis/2(q_axis) -> Qs/1
  sum_Ds/1 -> Switch_Axis/1(d)
  sum_Qs/1 -> Switch_Axis/2(q)
  cos/1 -> Data Type Duplicate/3, bcos/2, acos/2
  asin/1 -> sum_Qs/2
  bcos/1 -> sum_Qs/1
  bsin/1 -> sum_Ds/2
  acos/1 -> sum_Ds/1
  Alpha/1 -> Data Type Duplicate/1, acos/1, asin/1
  sine/1 -> bsin/2, asin/2, Data Type Duplicate/4

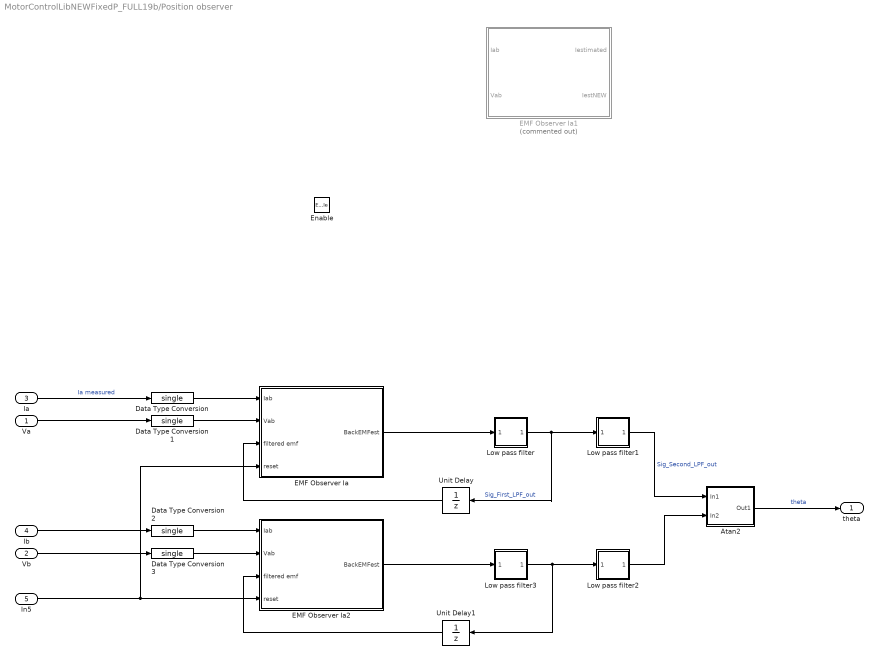
== system MotorControlLibNEWFixedP_FULL19b/Position observer ==
  Va : Inport
  Vb : Inport  Port=2
  Ia : Inport  Port=3
  Ib : Inport  Port=4
  In5 : Inport  Port=5
  Enable : EnablePort  StatesWhenEnabling=reset
  Atan2 : Subsystem
  Data Type Conversion{,1..3} (4 alike) : DataTypeConversion  OutDataTypeStr=single
  EMF Observer Ia : Subsystem  mask{Rs=EMFobsRS, Ld=EMFobsLdGain, P=Kp_Iab_EMFobs, I=Ki_Iab_EMFobs}
      mask prompts: Rs "Resistance"; Ld "Inductance"; P "Simulink:masks:ProportionalP_MP"; I "Simulink:masks:IntegralI_MP"
      mask TypeOptions Rs: DC Motor Model/Resistance/Gain
      mask TypeOptions Ld: DC Motor Model/Inductance/Gain
      mask TypeOptions P: PID Controller/P
      mask TypeOptions I: PID Controller/I
      mask DialogControl Container6 Prompt: PI Controller
      mask DialogControl P Prompt: Proportional (P):
      mask DialogControl I Prompt: Integral (I):
  EMF Observer Ia1 : Subsystem  Commented=on  mask{Rs=EMFobsRS, Ld=EMFobsLdGain, P=Kp_Iab_EMFobs, I=Ki_Iab_EMFobs}
      mask prompts: Rs "Resistance"; Ld "Inductance"; P "Simulink:masks:ProportionalP_MP"; I "Simulink:masks:IntegralI_MP"
      mask TypeOptions Rs: DC Motor Model/Resistance/Gain
      mask TypeOptions Ld: DC Motor Model/Inductance/Gain
      mask TypeOptions P: PID Controller/P
      mask TypeOptions I: PID Controller/I
      mask DialogControl Container6 Prompt: PI Controller
      mask DialogControl P Prompt: Proportional (P):
      mask DialogControl I Prompt: Integral (I):
  EMF Observer Ia2 : Subsystem  mask{Rs=EMFobsRS, Ld=EMFobsLdGain, P=Kp_Iab_EMFobs, I=Ki_Iab_EMFobs}
      mask prompts: Rs "Resistance"; Ld "Inductance"; P "Simulink:masks:ProportionalP_MP"; I "Simulink:masks:IntegralI_MP"
      mask TypeOptions Rs: DC Motor Model/Resistance/Gain
      mask TypeOptions Ld: DC Motor Model/Inductance/Gain
      mask TypeOptions P: PID Controller/P
      mask TypeOptions I: PID Controller/I
      mask DialogControl Container6 Prompt: PI Controller
      mask DialogControl P Prompt: Proportional (P):
      mask DialogControl I Prompt: Integral (I):
  Low pass filter : Subsystem  mask{Value=CuttOffFreq_c, Gain=250e-6}
      mask prompts: Value "CuttOff Freq."; Gain "Time interval"
      settings: AttributesFormatString=Integration constant %<Gain>
      mask TypeOptions Value: Constant/Value
      mask TypeOptions Gain: Gain/Gain
  Low pass filter1 : Subsystem  mask{Value=CuttOffFreq_c, Gain=250e-6}
      mask prompts: Value "CuttOff Freq."; Gain "Time interval"
      settings: AttributesFormatString=Integration constant %<Gain>
      mask TypeOptions Value: Constant/Value
      mask TypeOptions Gain: Gain/Gain
  Low pass filter2 : Subsystem  mask{Value=CuttOffFreq_c, Gain=250e-6}
      mask prompts: Value "CuttOff Freq."; Gain "Time interval"
      settings: AttributesFormatString=Integration constant %<Gain>
      mask TypeOptions Value: Constant/Value
      mask TypeOptions Gain: Gain/Gain
  Low pass filter3 : Subsystem  mask{Value=CuttOffFreq_c, Gain=250e-6}
      mask prompts: Value "CuttOff Freq."; Gain "Time interval"
      settings: AttributesFormatString=Integration constant %<Gain>
      mask TypeOptions Value: Constant/Value
      mask TypeOptions Gain: Gain/Gain
  Unit Delay : UnitDelay  SampleTime=-1  HasFrameUpgradeWarning=on
  Unit Delay1 : UnitDelay  SampleTime=-1  HasFrameUpgradeWarning=on
  theta : Outport
  wires:
  Atan2/1(Out1) -> theta/1  "theta"
  Va/1 -> Data Type Conversion1/1
  Ia/1 -> Data Type Conversion/1  "Ia measured"
  Vb/1 -> Data Type Conversion3/1
  Ib/1 -> Data Type Conversion2/1
  EMF Observer Ia/1(BackEMFest) -> Low pass filter/1(In1)
  Low pass filter/1(Output) -> Low pass filter1/1(In1), Unit Delay/1  "Sig_First_LPF_out"
  EMF Observer Ia2/1(BackEMFest) -> Low pass filter3/1(In1)
  Low pass filter3/1(Output) -> Low pass filter2/1(In1), Unit Delay1/1
  Low pass filter1/1(Output) -> Atan2/1(In1)  "Sig_Second_LPF_out"
  Low pass filter2/1(Output) -> Atan2/2(In2)
  Unit Delay/1 -> EMF Observer Ia/3(filtered emf)
  Unit Delay1/1 -> EMF Observer Ia2/3(filtered emf)
  In5/1 -> EMF Observer Ia/4(reset), EMF Observer Ia2/4(reset)
  Data Type Conversion/1 -> EMF Observer Ia/1(Iab)
  Data Type Conversion1/1 -> EMF Observer Ia/2(Vab)
  Data Type Conversion2/1 -> EMF Observer Ia2/1(Iab)
  Data Type Conversion3/1 -> EMF Observer Ia2/2(Vab)

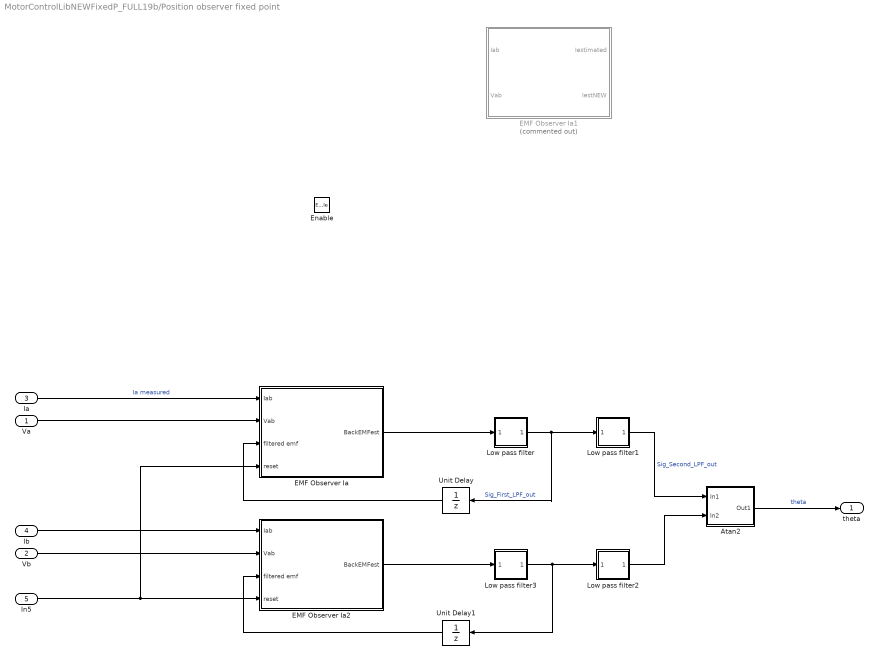
== system MotorControlLibNEWFixedP_FULL19b/Position observer fixed point ==
  Va : Inport
  Vb : Inport  Port=2
  Ia : Inport  Port=3
  Ib : Inport  Port=4
  In5 : Inport  Port=5
  Enable : EnablePort  StatesWhenEnabling=reset
  Atan2 : Subsystem
  EMF Observer Ia : Subsystem  mask{Rs=EMFobsRS, Ld=EMFobsLdGain, P=Kp_Iab_EMFobs, I=Ki_Iab_EMFobs}
      mask prompts: Rs "Resistance"; Ld "Inductance"; P "Simulink:masks:ProportionalP_MP"; I "Simulink:masks:IntegralI_MP"
      mask TypeOptions Rs: DC Motor Model/Resistance/Gain
      mask TypeOptions Ld: DC Motor Model/Inductance/Gain
      mask TypeOptions P: PID Controller/P
      mask TypeOptions I: PID Controller/I
      mask DialogControl Container6 Prompt: PI Controller
      mask DialogControl P Prompt: Proportional (P):
      mask DialogControl I Prompt: Integral (I):
  EMF Observer Ia1 : Subsystem  Commented=on  mask{Rs=EMFobsRS, Ld=EMFobsLdGain, P=Kp_Iab_EMFobs, I=Ki_Iab_EMFobs}
      mask prompts: Rs "Resistance"; Ld "Inductance"; P "Simulink:masks:ProportionalP_MP"; I "Simulink:masks:IntegralI_MP"
      mask TypeOptions Rs: DC Motor Model/Resistance/Gain
      mask TypeOptions Ld: DC Motor Model/Inductance/Gain
      mask TypeOptions P: PID Controller/P
      mask TypeOptions I: PID Controller/I
      mask DialogControl Container6 Prompt: PI Controller
      mask DialogControl P Prompt: Proportional (P):
      mask DialogControl I Prompt: Integral (I):
  EMF Observer Ia2 : Subsystem  mask{Rs=EMFobsRS, Ld=EMFobsLdGain, P=Kp_Iab_EMFobs, I=Ki_Iab_EMFobs}
      mask prompts: Rs "Resistance"; Ld "Inductance"; P "Simulink:masks:ProportionalP_MP"; I "Simulink:masks:IntegralI_MP"
      mask TypeOptions Rs: DC Motor Model/Resistance/Gain
      mask TypeOptions Ld: DC Motor Model/Inductance/Gain
      mask TypeOptions P: PID Controller/P
      mask TypeOptions I: PID Controller/I
      mask DialogControl Container6 Prompt: PI Controller
      mask DialogControl P Prompt: Proportional (P):
      mask DialogControl I Prompt: Integral (I):
  Low pass filter : Subsystem  mask{Value=CuttOffFreq_c, Gain=250e-6}
      mask prompts: Value "CuttOff Freq."; Gain "Time interval"
      settings: AttributesFormatString=Integration constant %<Gain>
      mask TypeOptions Value: Constant/Value
      mask TypeOptions Gain: Gain/Gain
  Low pass filter1 : Subsystem  mask{Value=CuttOffFreq_c, Gain=250e-6}
      mask prompts: Value "CuttOff Freq."; Gain "Time interval"
      settings: AttributesFormatString=Integration constant %<Gain>
      mask TypeOptions Value: Constant/Value
      mask TypeOptions Gain: Gain/Gain
  Low pass filter2 : Subsystem  mask{Value=CuttOffFreq_c, Gain=250e-6}
      mask prompts: Value "CuttOff Freq."; Gain "Time interval"
      settings: AttributesFormatString=Integration constant %<Gain>
      mask TypeOptions Value: Constant/Value
      mask TypeOptions Gain: Gain/Gain
  Low pass filter3 : Subsystem  mask{Value=CuttOffFreq_c, Gain=250e-6}
      mask prompts: Value "CuttOff Freq."; Gain "Time interval"
      settings: AttributesFormatString=Integration constant %<Gain>
      mask TypeOptions Value: Constant/Value
      mask TypeOptions Gain: Gain/Gain
  Unit Delay : UnitDelay  SampleTime=-1  HasFrameUpgradeWarning=on
  Unit Delay1 : UnitDelay  SampleTime=-1  HasFrameUpgradeWarning=on
  theta : Outport
  wires:
  Atan2/1(Out1) -> theta/1  "theta"
  Va/1 -> EMF Observer Ia/2(Vab)
  Ia/1 -> EMF Observer Ia/1(Iab)  "Ia measured"
  Vb/1 -> EMF Observer Ia2/2(Vab)
  Ib/1 -> EMF Observer Ia2/1(Iab)
  EMF Observer Ia/1(BackEMFest) -> Low pass filter/1(In1)
  Low pass filter/1(Output) -> Low pass filter1/1(In1), Unit Delay/1  "Sig_First_LPF_out"
  EMF Observer Ia2/1(BackEMFest) -> Low pass filter3/1(In1)
  Low pass filter3/1(Output) -> Low pass filter2/1(In1), Unit Delay1/1
  Low pass filter1/1(Output) -> Atan2/1(In1)  "Sig_Second_LPF_out"
  Low pass filter2/1(Output) -> Atan2/2(In2)
  Unit Delay/1 -> EMF Observer Ia/3(filtered emf)
  Unit Delay1/1 -> EMF Observer Ia2/3(filtered emf)
  In5/1 -> EMF Observer Ia/4(reset), EMF Observer Ia2/4(reset)

== system MotorControlLibNEWFixedP_FULL19b/Start up ==
  In1 : Inport
  In2 : Inport  Port=2
  Logic after motor is stoped : Subsystem
  Simulate start up Theta : Subsystem
  theta : Outport
  logic : Outport  Port=2
  wires:
  In1/1 -> Logic after motor is stoped/1(In1)
  Logic after motor is stoped/1(Out1) -> logic/1
  In2/1 -> Simulate start up Theta/1(In1)
  Simulate start up Theta/1(Out1) -> theta/1

== system MotorControlLibNEWFixedP_FULL19b/Calculate spin speed/2 * pi offset ==
  function : TriggerPort  TriggerType=function-call  VariantControl=Variant
  Constant : Constant  Value=2*pi  OutDataTypeStr=single
  Out1 : Outport
  wires:
  Constant/1 -> Out1/1

== system MotorControlLibNEWFixedP_FULL19b/Calculate spin speed/No offset ==
  function : TriggerPort  TriggerType=function-call  VariantControl=Variant
  Constant : Constant  Value=0  OutDataTypeStr=single
  Out1 : Outport
  wires:
  Constant/1 -> Out1/1

== system MotorControlLibNEWFixedP_FULL19b/Commented/Subsystem ==
  Clock : Inport
  function : TriggerPort  TriggerType=function-call  VariantControl=Variant
  Add2 : Sum  Inputs=+-
  Unit Conversion1 : UnitConversion  OutputType=Inherit: Inherit via back propagation
  Unit Delay : UnitDelay  SampleTime=-1  HasFrameUpgradeWarning=on
  dt : Outport
  wires:
  Add2/1 -> Unit Conversion1/1  "TimeMS"
  Unit Delay/1 -> Add2/2
  Clock/1 -> Unit Delay/1, Add2/1
  Unit Conversion1/1 -> dt/1  "Tsec"

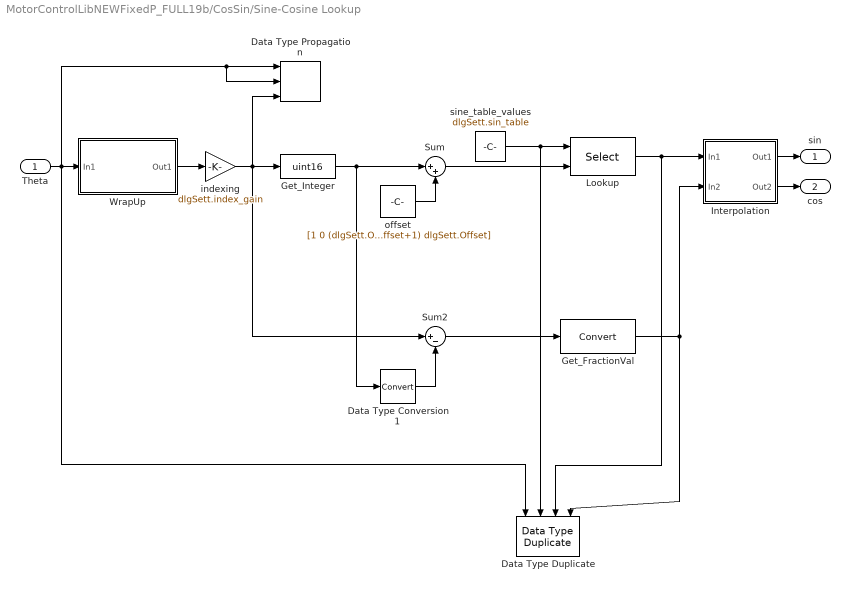
== system MotorControlLibNEWFixedP_FULL19b/CosSin/Sine-Cosine Lookup ==
  Theta : Inport
  Data Type Duplicate : DataTypeDuplicate  NumInputPorts=4
  Data Type Propagation : simulink/Signal Attributes/Data Type Propagation  PropDataType=fixdt(1, 16)  IfRefDouble=double  IfRefSingle=single  IsSigned=IsSigned1 or IsSigned2  NumBitsBase=max([NumBits1 NumBits2])  NumBitsMult=1  NumBitsAdd=0  NumBitsAllowFinal=1:128  PropScalingMode=Obtain via best precision  PropScaling=2^-10  ValuesUsedBestPrec=[0 dlgSett.index_gain]  SlopeBase=min([Slope1 Slope2])  SlopeMult=1  SlopeAdd=0  BiasBase=Bias1  BiasMult=1  BiasAdd=0
      settings: SourceProductBaseCode=SL
  Data Type Conversion1 : DataTypeConversion  RndMeth=Simplest
  Get_FractionVal : DataTypeConversion  RndMeth=Simplest
  Get_Integer : DataTypeConversion  OutDataTypeStr=uint16  RndMeth=Simplest
  Interpolation : Subsystem
  Lookup : Selector  IndexMode=Zero-based  InputPortWidth=dlgSett.size  IndexOptions=Index vector (port)  Indices=[1 3]  OutputSizes=1
  Sum : Sum  Inputs=|++  AccumDataTypeStr=uint32  OutDataTypeStr=uint32  RndMeth=Simplest
  Sum2 : Sum  Inputs=|+-  RndMeth=Simplest  OutDataTypeStr=Inherit: Same as first input
  WrapUp : Subsystem
  indexing : Gain  Gain=dlgSett.index_gain  OutDataTypeStr=Inherit: Inherit via back propagation  RndMeth=Simplest
  offset : Constant  Value=[1 0 (dlgSett.Offset+1) dlgSett.Offset]  OutDataTypeStr=int16  SampleTime=-1
  sine_table_values : Constant  Value=dlgSett.sin_table  OutDataTypeStr=Inherit: Inherit via back propagation  SampleTime=-1
  sin : Outport  VectorParamsAs1DForOutWhenUnconnected=off
  cos : Outport  Port=2  VectorParamsAs1DForOutWhenUnconnected=off
  wires:
  Interpolation/2(Out2) -> cos/1
  Interpolation/1(Out1) -> sin/1
  Sum/1 -> Lookup/2
  indexing/1 -> Sum2/1, Data Type Propagation/3, Get_Integer/1
  Data Type Conversion1/1 -> Sum2/2
  Get_Integer/1 -> Sum/1, Data Type Conversion1/1
  offset/1 -> Sum/2
  sine_table_values/1 -> Lookup/1, Data Type Duplicate/2
  Lookup/1 -> Interpolation/1(In1), Data Type Duplicate/3
  Sum2/1 -> Get_FractionVal/1
  Get_FractionVal/1 -> Data Type Duplicate/4, Interpolation/2(In2)
  Theta/1 -> Data Type Duplicate/1, WrapUp/1(In1), Data Type Propagation/2, Data Type Propagation/1
  WrapUp/1(Out1) -> indexing/1
